simulink model "VCMGCM1962020b_v2"  (R2020b)
settings: Solver=FixedStepDiscrete  StartTime=0.0  StopTime=10.0  FixedStep=0.005  RelTol=1e-3  EnableMultiTasking=on
PreLoadFcn:
  | try, model_open; catch, disp('Error occurred while executing model pre-load callback: model_open.m'); disp('Please assure that the MATLAB working directory is set to the model directory before opening.'); end
InitFcn:
  | try, model_open; catch, end
undefined symbols (not defined in the file): Bridge, GCM, H, raptor_get_param_eval, raptor_get_safe_string, raptor_xcp_function
libraries: Blocks_lib x1165, Raptor_lib x665, simulink x62, VCM_lib x5
(part 18 of 23)

== system VCMGCM1962020b_v2/Fgnd/Sensors/CAN/Inverter/EM3_DCV/EM3PhCur ==
  DiagEnbl : Inport
  Enable : EnablePort
  CANRxFieldSingleFloat : Subsystem  AncestorBlock=Blocks_lib/CANRxField  mask(CANRxField){typ='double', custom=off, custom_nam='---', custom_units='---'}
      mask prompts: typ "Field Data Type"; custom "Use Custom Name and Units (instead of from .dbc file)"; custom_nam "Custom Name"; custom_units "Custom Units"
      mask help:
      | To be used with the raptor_can_rxmsg block.
      |
      | By default, the field name/units will be inherited from the .dbc file. For Custom Name or Units, check the checkbox. To use the inherited name/units in the custom name/units, use the string '---' to inhereit. For example, to simply add a prefix, the custom name would be something like 'prefix_---'.
      mask init: same as VCMGCM1962020b_v2/Fgnd/Sensors/CAN/Inverter/EM2_InvTemp/EM2InvTemp/CANRxFieldSingleFloat
      mask Callback custom:
      | raptor_set_param_enable(gcb, 'custom_nam', strcmp(get_param(gcb, 'custom'), 'on'));
      | raptor_set_param_enable(gcb, 'custom_units', strcmp(get_param(gcb, 'custom'), 'on'));
      mask Display:
      | disp(['CAN Rx: Field\n' nam '\n' units ', ' typ]);
      | 
      | port_label('input', 1, 'In');
  CANRxMsgStatus : Blocks_lib/CANRxMsgStatus  samptime=samptime  custom=on  custom_nam='EM_PhaseA'  msgnam=EM_PhaseA
  Header : Blocks_lib/Header  width=Landscape  addtext=''
  raptor_can_rxmsg1 : Raptor_lib/CAN/raptor_can_rxmsg  canDefinition=struct('dbcFile', '20220526e_emDrive_NodeID_0x01.dbc','message', 'EM3','comment', '40ms','signals', {{'EM3_InverterDcV','EM3_PhaseAmpsRms'}},'enabled', [ 0 1;],'scaled', [ 1 1;],'canBus', 'bus','messageID', [ 897;],'idMask', [ 536870911;],'payloadMask', [],'payloadValue', [],'period', [ 0;],'mailbox', '''''','queueSize', [ 1;],'label', [ 1;],'ver', [ 2;],'showID', [ 0;],'showRaw', [ 0;],'fill', [ 0;],'editID', [ 0;],'signalOrder', [ 1;],'signalAscDes', [ 1;])  canBus=bus  mailbox=''  payloadMask=[]  payloadValue=[]  idMask=hex2dec('1FFFFFFF')  queueSize=1  showID=0  label=1  fill=0  id=897  showRaw=0  showAge=1  signalOrder=1  signalInfo={{struct('Name', 'EM3_InverterDcV','Startbit', [ 0;],'SignalSize', [ 32;],'ByteOrder', 'LittleEndian','ValueType', 'FLOAT32','Class', 'single','Signed', [ 1;],'Factor', [ 1;],'Offset', [ 0;],'Min', [ 0;],'Max', [ 0;],'Units', 'V','Comment', 'HW_Monitor__UDC','StartBit', [ 0;]),struct('Name', 'EM3_PhaseAmpsRms','Startbit', [ 0;],'SignalSize', [ 32;],'ByteOrder', 'LittleEndian','ValueType', 'FLOAT32','Class', 'single','Signed', [ 1;],'Factor', [ 1;],'Offset', [ 0;],'Min', [ 0;],'Max', [ 0;],'Units', 'A','Comment', 'HW_Monitor__Phase_Current','StartBit', [ 32;])}}
      settings: SourceProductName=Raptor
  MsgVld : Outport
  Out2 : Outport  Port=2
  wires:
  raptor_can_rxmsg1/2 -> CANRxFieldSingleFloat/1(In)  "EM3_PhaseAmpsRms"
  raptor_can_rxmsg1/1 -> CANRxMsgStatus/2  "Age"
  DiagEnbl/1 -> CANRxMsgStatus/1
  CANRxFieldSingleFloat/1(Out) -> Out2/1
  CANRxMsgStatus/1 -> MsgVld/1

== system VCMGCM1962020b_v2/Fgnd/Sensors/CAN/Inverter/EM4_Spd/EM4Spd ==
  note: TBC: This logic is to get around an issue with a divide by a very small number, which is not recognized as zero
  DiagEnbl : Inport
  Enable : EnablePort
  Abs : Abs
  Bus Creator : BusCreator  Inputs=2
  Bus Selector : BusSelector  OutputSignals=EM4_SpdActVld [Bool],EM4_SpdAct [rpm]
  CANRxFieldSingleFloat : Subsystem  AncestorBlock=Blocks_lib/CANRxField  mask(CANRxField){typ='double', custom=off, custom_nam='---', custom_units='---'}
      mask prompts: typ "Field Data Type"; custom "Use Custom Name and Units (instead of from .dbc file)"; custom_nam "Custom Name"; custom_units "Custom Units"
      mask help:
      | To be used with the raptor_can_rxmsg block.
      |
      | By default, the field name/units will be inherited from the .dbc file. For Custom Name or Units, check the checkbox. To use the inherited name/units in the custom name/units, use the string '---' to inhereit. For example, to simply add a prefix, the custom name would be something like 'prefix_---'.
      mask init: same as VCMGCM1962020b_v2/Fgnd/Sensors/CAN/Inverter/EM2_InvTemp/EM2InvTemp/CANRxFieldSingleFloat
      mask Callback custom:
      | raptor_set_param_enable(gcb, 'custom_nam', strcmp(get_param(gcb, 'custom'), 'on'));
      | raptor_set_param_enable(gcb, 'custom_units', strcmp(get_param(gcb, 'custom'), 'on'));
      mask Display:
      | disp(['CAN Rx: Field\n' nam '\n' units ', ' typ]);
      | 
      | port_label('input', 1, 'In');
  CANRxMsgStatus : Blocks_lib/CANRxMsgStatus  samptime=samptime  custom=on  custom_nam='EM4_Spd'  msgnam=EM4_Spd
  Compare To Constant : simulink/Logic and Bit Operations/Compare To Constant  relop=>  const=1  OutDataTypeStr=boolean
  Constant : Constant  Value=0
  Header : Blocks_lib/Header  width=Landscape  addtext=''
  Switch : Switch  Criteria=u2 > Threshold
  raptor_can_rxmsg1 : Raptor_lib/CAN/raptor_can_rxmsg  canDefinition=struct('dbcFile', '20220526e_emDrive_NodeID_0x01.dbc','message', 'EM4','comment', '20ms','signals', {{'EM4_SpdAct','EM4_TorqAct'}},'enabled', [ 1 0;],'scaled', [ 1 1;],'canBus', 'bus','messageID', [ 641;],'idMask', [ 536870911;],'payloadMask', [],'payloadValue', [],'period', [ 0;],'mailbox', '''''','queueSize', [ 1;],'label', [ 1;],'ver', [ 2;],'showID', [ 0;],'showRaw', [ 0;],'fill', [ 0;],'editID', [ 0;],'signalOrder', [ 1;],'signalAscDes', [ 1;])  canBus=bus  mailbox=''  payloadMask=[]  payloadValue=[]  idMask=hex2dec('1FFFFFFF')  queueSize=1  showID=0  label=1  fill=0  id=641  showRaw=0  showAge=1  signalOrder=1  signalInfo={{struct('Name', 'EM4_TorqAct','Startbit', [ 0;],'SignalSize', [ 32;],'ByteOrder', 'LittleEndian','ValueType', 'FLOAT32','Class', 'single','Signed', [ 1;],'Factor', [ 1;],'Offset', [ 0;],'Min', [ 0;],'Max', [ 0;],'Units', 'Nm','Comment', 'Ctrl_Gen_Stat__Tact','StartBit', [ 0;]),struct('Name', 'EM4_SpdAct','Startbit', [ 0;],'SignalSize', [ 32;],'ByteOrder', 'LittleEndian','ValueType', 'FLOAT32','Class', 'single','Signed', [ 1;],'Factor', [ 1;],'Offset', [ 0;],'Min', [ 0;],'Max', [ 0;],'Units', 'rpm','Comment', 'Ctrl_Gen_Stat__RPMact','StartBit', [ 32;])}}
      settings: SourceProductName=Raptor
  MsgVld : Outport
  Out2 : Outport  Port=2
  wires:
  raptor_can_rxmsg1/2 -> CANRxFieldSingleFloat/1(In)  "EM4_SpdAct"
  raptor_can_rxmsg1/1 -> CANRxMsgStatus/2  "Age"
  DiagEnbl/1 -> CANRxMsgStatus/1
  CANRxMsgStatus/1 -> MsgVld/1
  Constant/1 -> Switch/3
  Abs/1 -> Compare To Constant/1
  Compare To Constant/1 -> Switch/2
  CANRxFieldSingleFloat/1(Out) -> Bus Selector/1
  Bus Selector/2 -> Switch/1, Abs/1  "<EM4_SpdAct [rpm]>"
  Bus Creator/1 -> Out2/1  "EM4_SpdAct"
  Bus Selector/1 -> Bus Creator/1  "<EM4_SpdActVld [Bool]>"
  Switch/1 -> Bus Creator/2  "EM4_SpdAct [rpm]"

== system VCMGCM1962020b_v2/Fgnd/Sensors/CAN/Inverter/EM4_Spd/EM4Torq ==
  DiagEnbl : Inport
  Enable : EnablePort
  CANRxFieldSingleFloat : Subsystem  AncestorBlock=Blocks_lib/CANRxField  mask(CANRxField){typ='double', custom=off, custom_nam='---', custom_units='---'}
      mask prompts: typ "Field Data Type"; custom "Use Custom Name and Units (instead of from .dbc file)"; custom_nam "Custom Name"; custom_units "Custom Units"
      mask help:
      | To be used with the raptor_can_rxmsg block.
      |
      | By default, the field name/units will be inherited from the .dbc file. For Custom Name or Units, check the checkbox. To use the inherited name/units in the custom name/units, use the string '---' to inhereit. For example, to simply add a prefix, the custom name would be something like 'prefix_---'.
      mask init: same as VCMGCM1962020b_v2/Fgnd/Sensors/CAN/Inverter/EM2_InvTemp/EM2InvTemp/CANRxFieldSingleFloat
      mask Callback custom:
      | raptor_set_param_enable(gcb, 'custom_nam', strcmp(get_param(gcb, 'custom'), 'on'));
      | raptor_set_param_enable(gcb, 'custom_units', strcmp(get_param(gcb, 'custom'), 'on'));
      mask Display:
      | disp(['CAN Rx: Field\n' nam '\n' units ', ' typ]);
      | 
      | port_label('input', 1, 'In');
  CANRxMsgStatus : Blocks_lib/CANRxMsgStatus  samptime=samptime  custom=on  custom_nam='EM4_Trq'  msgnam=EM4_Trq
  Header : Blocks_lib/Header  width=Landscape  addtext=''
  raptor_can_rxmsg1 : Raptor_lib/CAN/raptor_can_rxmsg  canDefinition=struct('dbcFile', '20220526e_emDrive_NodeID_0x01.dbc','message', 'EM4','comment', '20ms','signals', {{'EM4_SpdAct','EM4_TorqAct'}},'enabled', [ 0 1;],'scaled', [ 1 1;],'canBus', 'bus','messageID', [ 641;],'idMask', [ 536870911;],'payloadMask', [],'payloadValue', [],'period', [ 0;],'mailbox', '''''','queueSize', [ 1;],'label', [ 1;],'ver', [ 2;],'showID', [ 0;],'showRaw', [ 0;],'fill', [ 0;],'editID', [ 0;],'signalOrder', [ 1;],'signalAscDes', [ 1;])  canBus=bus  mailbox=''  payloadMask=[]  payloadValue=[]  idMask=hex2dec('1FFFFFFF')  queueSize=1  showID=0  label=1  fill=0  id=641  showRaw=0  showAge=1  signalOrder=1  signalInfo={{struct('Name', 'EM4_TorqAct','Startbit', [ 0;],'SignalSize', [ 32;],'ByteOrder', 'LittleEndian','ValueType', 'FLOAT32','Class', 'single','Signed', [ 1;],'Factor', [ 1;],'Offset', [ 0;],'Min', [ 0;],'Max', [ 0;],'Units', 'Nm','Comment', 'Ctrl_Gen_Stat__Tact','StartBit', [ 0;]),struct('Name', 'EM4_SpdAct','Startbit', [ 0;],'SignalSize', [ 32;],'ByteOrder', 'LittleEndian','ValueType', 'FLOAT32','Class', 'single','Signed', [ 1;],'Factor', [ 1;],'Offset', [ 0;],'Min', [ 0;],'Max', [ 0;],'Units', 'rpm','Comment', 'Ctrl_Gen_Stat__RPMact','StartBit', [ 32;])}}
      settings: SourceProductName=Raptor
  MsgVld : Outport
  Out2 : Outport  Port=2
  wires:
  raptor_can_rxmsg1/2 -> CANRxFieldSingleFloat/1(In)  "EM4_TorqAct"
  raptor_can_rxmsg1/1 -> CANRxMsgStatus/2  "Age"
  DiagEnbl/1 -> CANRxMsgStatus/1
  CANRxFieldSingleFloat/1(Out) -> Out2/1
  CANRxMsgStatus/1 -> MsgVld/1

== system VCMGCM1962020b_v2/Fgnd/Sensors/CAN/Other/A//C Compressor/ACCSTATUS2 ==
  DiagEnbl : Inport
  Bus Creator : BusCreator  Inputs=7
  CANRxField : Blocks_lib/CANRxField  typ='boolean'  custom=on  custom_nam=[nam '---']  custom_units='---'
  CANRxField1 : Blocks_lib/CANRxField  typ='boolean'  custom=on  custom_nam=[nam '---']  custom_units='---'
  CANRxField2 : Blocks_lib/CANRxField  typ='boolean'  custom=on  custom_nam=[nam '---']  custom_units='---'
  CANRxField3 : Blocks_lib/CANRxField  typ='double'  custom=on  custom_nam=[nam '---']  custom_units='---'
  CANRxField4 : Blocks_lib/CANRxField  typ='double'  custom=on  custom_nam=[nam '---']  custom_units='---'
  CANRxField5 : Blocks_lib/CANRxField  typ='double'  custom=on  custom_nam=[nam '---']  custom_units='---'
  CANRxMsgStatus : Blocks_lib/CANRxMsgStatus  samptime=samptime  custom=on  custom_nam=[nam '---']  msgnam=ACCSTATUS2
  Header : Blocks_lib/Header  width=Landscape  addtext=''
  raptor_can_rxmsg : Raptor_lib/CAN/raptor_can_rxmsg  canDefinition=struct('dbcFile', 'ACCompressor_MitsubishiEV36BNx.dbc','message', 'STATUS2','comment', '','signals', {{'IGBTTempV','HVInputV','BoardTempV','BoardTemp','HVInput','IGBTTemp'}},'enabled', [ 1 1 1 1 1 1;],'scaled', [ 1 1 1 1 1 1;],'canBus', 'bus','messageID', [ 141598791;],'idMask', [ 536870911;],'payloadMask', [],'payloadValue', [],'period', [ 0;],'mailbox', '''''','queueSize', [ 1;],'label', [ 1;],'ver', [ 2;],'showID', [ 0;],'showRaw', [ 0;],'fill', [ 0;],'editID', [ 0;],'signalOrder', [ 3;],'signalAscDes', [ 1;])  canBus=bus  mailbox=''  payloadMask=[]  payloadValue=[]  idMask=hex2dec('1FFFFFFF')  queueSize=1  showID=0  label=1  fill=0  id=141598791  showRaw=0  showAge=1  signalOrder=3  signalInfo={{struct('Name', 'IGBTTempV','Startbit', [ 0;],'SignalSize', [ 1;],'ByteOrder', 'LittleEndian','ValueType', 'UNSIGNED','Class', 'uint8','Signed', [ 0;],'Factor', [ 1;],'Offset', [ 0;],'Min', [ 0;],'Max', [ 1;],'Units', '','Comment', '','StartBit', [ 2;]),struct('Name', 'HVInputV','Startbit', [ 0;],'SignalSize', [ 1;],'ByteOrder', 'LittleEndian','ValueType', 'UNSIGNED','Class', 'uint8','Signed', [ 0;],'Factor', [ 1;],'Offset', [ 0;],'Min', [ 0;],'Max', [ 1;],'Units', '','Comment', '','StartBit', [ 1;]),struct('Name', 'BoardTempV','Startbit', [ 0;],'SignalSize', [ 1;],'ByteOrder', 'LittleEndian','ValueType', 'UNSIGNED','Class', 'uint8','Signed', [ 0;],'Factor', [ 1;],'Offset', [ 0;],'Min', [ 0;],'Max', [ 1;],'Units', '','Comment', '','StartBit', [ 0;]),struct('Name', 'BoardTemp','Startbit', [ 0;],'SignalSize', [ 8;],'ByteOrder', 'LittleEndian','ValueType', 'UNSIGNED','Class', 'uint8','Signed', [ 0;],'Factor', [ 1;],'Offset', [ -40;],'Min', [ -40;],'Max', [ 215;],'Units', 'degC','Comment', '','StartBit', [ 8;]),struct('Name', 'HVInput','Startbit', [ 0;],'SignalSize', [ 8;],'ByteOrder', 'LittleEndian','ValueType', 'UNSIGNED','Class', 'uint8','Signed', [ 0;],'Factor', [ 4;],'Offset', [ 0;],'Min', [ 0;],'Max', [ 1020;],'Units', 'Volts','Comment', '','StartBit', [ 16;]),struct('Name', 'IGBTTemp','Startbit', [ 0;],'SignalSize', [ 8;],'ByteOrder', 'LittleEndian','ValueType', 'UNSIGNED','Class', 'uint8','Signed', [ 0;],'Factor', [ 1;],'Offset', [ -40;],'Min', [ -40;],'Max', [ 215;],'Units', 'degC','Comment', '','StartBit', [ 24;])}}
      settings: SourceProductName=Raptor
  Data : Outport  VectorParamsAs1DForOutWhenUnconnected=off
  wires:
  raptor_can_rxmsg/1 -> CANRxMsgStatus/2  "Age"
  DiagEnbl/1 -> CANRxMsgStatus/1
  CANRxMsgStatus/1 -> Bus Creator/1
  CANRxField/1 -> Bus Creator/2
  raptor_can_rxmsg/3 -> CANRxField1/1  "HVInputV"
  raptor_can_rxmsg/2 -> CANRxField/1  "IGBTTempV"
  Bus Creator/1 -> Data/1  "MsgName"
  raptor_can_rxmsg/4 -> CANRxField2/1  "BoardTempV"
  raptor_can_rxmsg/5 -> CANRxField3/1  "BoardTemp"
  raptor_can_rxmsg/6 -> CANRxField4/1  "HVInput"
  raptor_can_rxmsg/7 -> CANRxField5/1  "IGBTTemp"
  CANRxField1/1 -> Bus Creator/3
  CANRxField2/1 -> Bus Creator/4
  CANRxField3/1 -> Bus Creator/5
  CANRxField4/1 -> Bus Creator/6
  CANRxField5/1 -> Bus Creator/7

== system VCMGCM1962020b_v2/Fgnd/Sensors/CAN/Other/A//C Compressor/MsgName ==
  DiagEnbl : Inport
  Bus Creator : BusCreator  Inputs=10
  CANRxField{,2..4} (4 alike) : Blocks_lib/CANRxField  typ='boolean'  custom=on  custom_nam=[nam '---']  custom_units='---'
  CANRxField1 : Blocks_lib/CANRxField  typ='uint8'  custom=on  custom_nam=[nam '---']  custom_units='---'
  CANRxField5 : Blocks_lib/CANRxField  typ='double'  custom=on  custom_nam=[nam '---']  custom_units='---'
  CANRxField6 : Blocks_lib/CANRxField  typ='double'  custom=on  custom_nam=[nam '---']  custom_units='---'
  CANRxField7 : Blocks_lib/CANRxField  typ='double'  custom=on  custom_nam=[nam '---']  custom_units='---'
  CANRxField8 : Blocks_lib/CANRxField  typ='uint8'  custom=on  custom_nam=[nam '---']  custom_units='---'
  CANRxMsgStatus : Blocks_lib/CANRxMsgStatus  samptime=samptime  custom=on  custom_nam=[nam '---']  msgnam=ACCSTATUS1
  Header : Blocks_lib/Header  width=Landscape  addtext=''
  raptor_can_rxmsg : Raptor_lib/CAN/raptor_can_rxmsg  canDefinition=struct('dbcFile', 'ACCompressor_MitsubishiEV36BNx.dbc','message', 'STATUS1','comment', '','signals', {{'ElecCurrV','Stat','ElecPwrV','SpdIncrReq','SpdV','ElecPwr','Spd','ElecCurr','FltStat'}},'enabled', [ 1 1 1 1 1 1 1 1 1;],'scaled', [ 1 1 1 1 1 1 1 1 1;],'canBus', 'bus','messageID', [ 141074503;],'idMask', [ 536870911;],'payloadMask', [],'payloadValue', [],'period', [ 0;],'mailbox', '''''','queueSize', [ 1;],'label', [ 1;],'ver', [ 2;],'showID', [ 0;],'showRaw', [ 0;],'fill', [ 0;],'editID', [ 0;],'signalOrder', [ 3;],'signalAscDes', [ 1;])  canBus=bus  mailbox=''  payloadMask=[]  payloadValue=[]  idMask=hex2dec('1FFFFFFF')  queueSize=1  showID=0  label=1  fill=0  id=141074503  showRaw=0  showAge=1  signalOrder=3  signalInfo={{struct('Name', 'ElecCurrV','Startbit', [ 0;],'SignalSize', [ 1;],'ByteOrder', 'LittleEndian','ValueType', 'UNSIGNED','Class', 'uint8','Signed', [ 0;],'Factor', [ 1;],'Offset', [ 0;],'Min', [ 0;],'Max', [ 1;],'Units', '','Comment', '','StartBit', [ 7;]),struct('Name', 'Stat','Startbit', [ 0;],'SignalSize', [ 4;],'ByteOrder', 'LittleEndian','ValueType', 'UNSIGNED','Class', 'uint8','Signed', [ 0;],'Factor', [ 1;],'Offset', [ 0;],'Min', [ 0;],'Max', [ 2;],'Units', '','Comment', '','StartBit', [ 3;]),struct('Name', 'ElecPwrV','Startbit', [ 0;],'SignalSize', [ 1;],'ByteOrder', 'LittleEndian','ValueType', 'UNSIGNED','Class', 'uint8','Signed', [ 0;],'Factor', [ 1;],'Offset', [ 0;],'Min', [ 0;],'Max', [ 0;],'Units', '','Comment', '','StartBit', [ 2;]),struct('Name', 'SpdIncrReq','Startbit', [ 0;],'SignalSize', [ 1;],'ByteOrder', 'LittleEndian','ValueType', 'UNSIGNED','Class', 'uint8','Signed', [ 0;],'Factor', [ 1;],'Offset', [ 0;],'Min', [ 0;],'Max', [ 1;],'Units', '','Comment', '','StartBit', [ 1;]),struct('Name', 'SpdV','Startbit', [ 0;],'SignalSize', [ 1;],'ByteOrder', 'LittleEndian','ValueType', 'UNSIGNED','Class', 'uint8','Signed', [ 0;],'Factor', [ 1;],'Offset', [ 0;],'Min', [ 0;],'Max', [ 1;],'Units', '','Comment', '','StartBit', [ 0;]),struct('Name', 'ElecPwr','Startbit', [ 0;],'SignalSize', [ 8;],'ByteOrder', 'LittleEndian','ValueType', 'UNSIGNED','Class', 'uint8','Signed', [ 0;],'Factor', [ 40;],'Offset', [ 0;],'Min', [ 0;],'Max', [ 10200;],'Units', 'Watts','Comment', '','StartBit', [ 8;]),struct('Name', 'Spd','Startbit', [ 0;],'SignalSize', [ 14;],'ByteOrder', 'BigEndian','ValueType', 'UNSIGNED','Class', 'uint16','Signed', [ 0;],'Factor', [ 1;],'Offset', [ 0;],'Min', [ 0;],'Max', [ 16383;],'Units', 'RPM','Comment', '','StartBit', [ 24;]),struct('Name', 'ElecCurr','Startbit', [ 0;],'SignalSize', [ 8;],'ByteOrder', 'LittleEndian','ValueType', 'UNSIGNED','Class', 'uint8','Signed', [ 0;],'Factor', [ 0.2;],'Offset', [ 0;],'Min', [ 0;],'Max', [ 51;],'Units', 'Amps','Comment', '','StartBit', [ 32;]),struct('Name', 'FltStat','Startbit', [ 0;],'SignalSize', [ 4;],'ByteOrder', 'LittleEndian','ValueType', 'UNSIGNED','Class', 'uint8','Signed', [ 0;],'Factor', [ 1;],'Offset', [ 0;],'Min', [ 0;],'Max', [ 6;],'Units', '','Comment', '','StartBit', [ 40;])}}
      settings: SourceProductName=Raptor
  Data : Outport  VectorParamsAs1DForOutWhenUnconnected=off
  wires:
  raptor_can_rxmsg/1 -> CANRxMsgStatus/2  "Age"
  DiagEnbl/1 -> CANRxMsgStatus/1
  CANRxMsgStatus/1 -> Bus Creator/1
  CANRxField/1 -> Bus Creator/2
  raptor_can_rxmsg/3 -> CANRxField1/1  "Stat"
  raptor_can_rxmsg/2 -> CANRxField/1  "ElecCurrV"
  Bus Creator/1 -> Data/1  "MsgName"
  raptor_can_rxmsg/4 -> CANRxField2/1  "ElecPwrV"
  raptor_can_rxmsg/5 -> CANRxField3/1  "SpdIncrReq"
  raptor_can_rxmsg/6 -> CANRxField4/1  "SpdV"
  raptor_can_rxmsg/7 -> CANRxField5/1  "ElecPwr"
  raptor_can_rxmsg/8 -> CANRxField6/1  "Spd"
  raptor_can_rxmsg/9 -> CANRxField7/1  "ElecCurr"
  raptor_can_rxmsg/10 -> CANRxField8/1  "FltStat"
  CANRxField1/1 -> Bus Creator/3
  CANRxField2/1 -> Bus Creator/4
  CANRxField3/1 -> Bus Creator/5
  CANRxField4/1 -> Bus Creator/6
  CANRxField5/1 -> Bus Creator/7
  CANRxField6/1 -> Bus Creator/8
  CANRxField7/1 -> Bus Creator/9
  CANRxField8/1 -> Bus Creator/10

== system VCMGCM1962020b_v2/Fgnd/Sensors/CAN/Other/BCM/BCMAMB ==
  DiagEnbl : Inport
  Bus Creator : BusCreator  Inputs=3
  CANRxField : Blocks_lib/CANRxField  typ='double'  custom=off  custom_nam=[nam '---']  custom_units='---'
  CANRxField1 : Blocks_lib/CANRxField  typ='double'  custom=off  custom_nam=[nam '---']  custom_units='---'
  CANRxMsgStatus : Blocks_lib/CANRxMsgStatus  samptime=samptime  custom=on  custom_nam=[nam '---']  msgnam=BCMAMB
  Header : Blocks_lib/Header  width=Landscape  addtext=''
  raptor_can_rxmsg : Raptor_lib/CAN/raptor_can_rxmsg  canDefinition=struct('dbcFile', 'BCM_dbc_file_rev_9.1.dbc','message', 'AMB','comment', '','signals', {{'Amb_Air_Temp','Cab_Temp'}},'enabled', [ 1 1;],'scaled', [ 1 1;],'canBus', 'bus','messageID', [ 419362081;],'idMask', [ 536870911;],'payloadMask', [],'payloadValue', [],'period', [ 0;],'mailbox', '[]','queueSize', [ 1;],'label', [ 1;],'ver', [ 2;],'showID', [ 0;],'showRaw', [ 0;],'fill', [ 0;],'editID', [ 0;],'signalOrder', [ 3;],'signalAscDes', [ 1;])  canBus=bus  mailbox=[]  payloadMask=[]  payloadValue=[]  idMask=hex2dec('1FFFFFFF')  queueSize=1  showID=0  label=1  fill=0  id=419362081  showRaw=0  showAge=1  signalOrder=3  signalInfo={{struct('Name', 'Amb_Air_Temp','Startbit', [ 0;],'SignalSize', [ 16;],'ByteOrder', 'LittleEndian','ValueType', 'UNSIGNED','Class', 'uint16','Signed', [ 0;],'Factor', [ 0.03125;],'Offset', [ -273;],'Min', [ -273;],'Max', [ 1734.97;],'Units', 'C','Comment', '','StartBit', [ 24;]),struct('Name', 'Cab_Temp','Startbit', [ 0;],'SignalSize', [ 16;],'ByteOrder', 'LittleEndian','ValueType', 'UNSIGNED','Class', 'uint16','Signed', [ 0;],'Factor', [ 0.03125;],'Offset', [ -273;],'Min', [ -273;],'Max', [ 1734.97;],'Units', 'C','Comment', '','StartBit', [ 8;])}}
      settings: SourceProductName=Raptor
  Data : Outport  VectorParamsAs1DForOutWhenUnconnected=off
  wires:
  raptor_can_rxmsg/3 -> CANRxField1/1  "Cab_Temp"
  Bus Creator/1 -> Data/1  "BCMAMB"
  raptor_can_rxmsg/2 -> CANRxField/1  "Amb_Air_Temp"
  CANRxMsgStatus/1 -> Bus Creator/1
  CANRxField/1 -> Bus Creator/2
  CANRxField1/1 -> Bus Creator/3
  DiagEnbl/1 -> CANRxMsgStatus/1
  raptor_can_rxmsg/1 -> CANRxMsgStatus/2  "Age"

== system VCMGCM1962020b_v2/Fgnd/Sensors/CAN/Other/BCM/BCMCab_Mssg1 ==
  DiagEnbl : Inport
  Bus Creator : BusCreator  Inputs=2
  CANRxField : Blocks_lib/CANRxField  typ='uint8'  custom=off  custom_nam=[nam '---']  custom_units='---'
  CANRxMsgStatus : Blocks_lib/CANRxMsgStatus  samptime=samptime  custom=on  custom_nam=[nam '---']  msgnam=BCMCab_Mssg1
  Header : Blocks_lib/Header  width=Landscape  addtext=''
  raptor_can_rxmsg : Raptor_lib/CAN/raptor_can_rxmsg  canDefinition=struct('dbcFile', 'BCM_dbc_file_rev_9.1.dbc','message', 'Cab_Mssg1','comment', '','signals', {{'Seatbelt_Switch'}},'enabled', [ 1;],'scaled', [ 1;],'canBus', 'bus','messageID', [ 417333281;],'idMask', [ 536870911;],'payloadMask', [],'payloadValue', [],'period', [ 0;],'mailbox', '[]','queueSize', [ 1;],'label', [ 1;],'ver', [ 2;],'showID', [ 0;],'showRaw', [ 0;],'fill', [ 0;],'editID', [ 0;],'signalOrder', [ 3;],'signalAscDes', [ 1;])  canBus=bus  mailbox=[]  payloadMask=[]  payloadValue=[]  idMask=hex2dec('1FFFFFFF')  queueSize=1  showID=0  label=1  fill=0  id=417333281  showRaw=0  showAge=1  signalOrder=3  signalInfo={{struct('Name', 'Seatbelt_Switch','Startbit', [ 0;],'SignalSize', [ 2;],'ByteOrder', 'LittleEndian','ValueType', 'UNSIGNED','Class', 'uint8','Signed', [ 0;],'Factor', [ 1;],'Offset', [ 0;],'Min', [ 0;],'Max', [ 3;],'Units', 'enum','Comment', '','StartBit', [ 30;])}}
      settings: SourceProductName=Raptor
  Data : Outport  VectorParamsAs1DForOutWhenUnconnected=off
  wires:
  Bus Creator/1 -> Data/1  "BCMCab_Mssg1"
  raptor_can_rxmsg/2 -> CANRxField/1  "Seatbelt_Switch"
  CANRxMsgStatus/1 -> Bus Creator/1
  CANRxField/1 -> Bus Creator/2
  DiagEnbl/1 -> CANRxMsgStatus/1
  raptor_can_rxmsg/1 -> CANRxMsgStatus/2  "Age"

== system VCMGCM1962020b_v2/Fgnd/Sensors/CAN/Other/BCM/CCVS1_BCM ==
  DiagEnbl : Inport
  Bus Creator : BusCreator  Inputs=2
  CANRxField : Blocks_lib/CANRxField  typ='uint8'  custom=off  custom_nam=[nam '---']  custom_units='---'
  CANRxMsgStatus : Blocks_lib/CANRxMsgStatus  samptime=samptime  custom=off  custom_nam=[nam '---']  msgnam=CCVS1_BCM
  Header : Blocks_lib/Header  width=Landscape  addtext=''
  raptor_can_rxmsg : Raptor_lib/CAN/raptor_can_rxmsg  canDefinition=struct('dbcFile', 'BCM_dbc_file_rev_9.1.dbc','message', 'CCVS1_BCM','comment', '','signals', {{'Parking_Brak_Switch'}},'enabled', [ 1;],'scaled', [ 1;],'canBus', 'bus','messageID', [ 419361057;],'idMask', [ 536870911;],'payloadMask', [],'payloadValue', [],'period', [ 0;],'mailbox', '[]','queueSize', [ 1;],'label', [ 1;],'ver', [ 2;],'showID', [ 0;],'showRaw', [ 0;],'fill', [ 0;],'editID', [ 0;],'signalOrder', [ 3;],'signalAscDes', [ 1;])  canBus=bus  mailbox=[]  payloadMask=[]  payloadValue=[]  idMask=hex2dec('1FFFFFFF')  queueSize=1  showID=0  label=1  fill=0  id=419361057  showRaw=0  showAge=1  signalOrder=3  signalInfo={{struct('Name', 'Parking_Brak_Switch','Startbit', [ 0;],'SignalSize', [ 2;],'ByteOrder', 'LittleEndian','ValueType', 'UNSIGNED','Class', 'uint8','Signed', [ 0;],'Factor', [ 1;],'Offset', [ 0;],'Min', [ 0;],'Max', [ 3;],'Units', 'enum','Comment', '','StartBit', [ 0;])}}
      settings: SourceProductName=Raptor
  Data : Outport  VectorParamsAs1DForOutWhenUnconnected=off
  wires:
  Bus Creator/1 -> Data/1  "CCVS1_BCM"
  raptor_can_rxmsg/2 -> CANRxField/1  "Parking_Brak_Switch"
  CANRxMsgStatus/1 -> Bus Creator/1
  CANRxField/1 -> Bus Creator/2
  DiagEnbl/1 -> CANRxMsgStatus/1
  raptor_can_rxmsg/1 -> CANRxMsgStatus/2  "Age"

== system VCMGCM1962020b_v2/Fgnd/Sensors/CAN/Other/BCM1/DisplayTG1 ==
  DiagEnbl : Inport
  Bus Creator : BusCreator  Inputs=2
  CANRxField : Blocks_lib/CANRxField  typ='double'  custom=off  custom_nam=[nam '---']  custom_units='---'
  CANRxMsgStatus : Blocks_lib/CANRxMsgStatus  samptime=samptime  custom=on  custom_nam=[nam '---']  msgnam=DisplayTG1
  Header : Blocks_lib/Header  width=Landscape  addtext=''
  raptor_can_rxmsg : Raptor_lib/CAN/raptor_can_rxmsg  canDefinition=struct('dbcFile', 'Drivers_Disp_dbc_file_v5.0.dbc','message', 'TG1','comment', '','signals', {{'Trip_Reset'}},'enabled', [ 1;],'scaled', [ 1;],'canBus', 'bus','messageID', [ 417202430;],'idMask', [ 536870911;],'payloadMask', [],'payloadValue', [],'period', [ 0;],'mailbox', '[]','queueSize', [ 1;],'label', [ 1;],'ver', [ 2;],'showID', [ 0;],'showRaw', [ 0;],'fill', [ 0;],'editID', [ 0;],'signalOrder', [ 3;],'signalAscDes', [ 1;])  canBus=bus  mailbox=[]  payloadMask=[]  payloadValue=[]  idMask=hex2dec('1FFFFFFF')  queueSize=1  showID=0  label=1  fill=0  id=417202430  showRaw=0  showAge=1  signalOrder=3  signalInfo={{struct('Name', 'Trip_Reset','Startbit', [ 0;],'SignalSize', [ 2;],'ByteOrder', 'LittleEndian','ValueType', 'UNSIGNED','Class', 'uint8','Signed', [ 0;],'Factor', [ 1;],'Offset', [ 0;],'Min', [ 0;],'Max', [ 3;],'Units', 'enum','Comment', '','StartBit', [ 0;])}}
      settings: SourceProductName=Raptor
  Data : Outport  VectorParamsAs1DForOutWhenUnconnected=off
  wires:
  Bus Creator/1 -> Data/1  "DisplayTG1"
  raptor_can_rxmsg/2 -> CANRxField/1  "Trip_Reset"
  CANRxMsgStatus/1 -> Bus Creator/1
  CANRxField/1 -> Bus Creator/2
  DiagEnbl/1 -> CANRxMsgStatus/1
  raptor_can_rxmsg/1 -> CANRxMsgStatus/2  "Age"

== system VCMGCM1962020b_v2/Fgnd/Sensors/CAN/Other/Charge Port DC Voltage Sensor/cs_ivt_msg_result_voltage_ch1 ==
  DiagEnbl : Inport
  Bus Creator : BusCreator  Inputs=8
  CANRxField{,1,5..6} (4 alike) : Blocks_lib/CANRxField  typ='boolean'  custom=off  custom_nam='---'  custom_units='---'
  CANRxField2 : Blocks_lib/CANRxField  typ='double'  custom=off  custom_nam='---'  custom_units='---'
  CANRxField3 : Blocks_lib/CANRxField  typ='uint8'  custom=off  custom_nam='---'  custom_units='---'
  CANRxField4 : Blocks_lib/CANRxField  typ='uint8'  custom=off  custom_nam='---'  custom_units='---'
  CANRxMsgStatus : Blocks_lib/CANRxMsgStatus  samptime=samptime  custom=off  custom_nam='Name'  msgnam=cs_ivt_msg_result_voltage_ch1
  Header : Blocks_lib/Header  width=Landscape  addtext=''
  raptor_can_rxmsg : Raptor_lib/CAN/raptor_can_rxmsg  canDefinition=struct('dbcFile', 'ivt_current_sensor.dbc','message', 'cs_ivt_msg_result_voltage_ch1','comment', '','signals', {{'result_volt_ch1_channel_error','result_volt_ch1_meas_error','result_volt_ch1_meas_value','result_volt_ch1_msg_count','result_volt_ch1_mux_id','result_volt_ch1_system_error','result_volt_ch1_ocs'}},'enabled', [ 1 1 1 1 1 1 1;],'scaled', [ 1 1 1 1 1 1 1;],'canBus', 'bus','messageID', [ 1314;],'idMask', [ 536870911;],'payloadMask', [],'payloadValue', [],'period', [ 0;],'mailbox', '''''','queueSize', [ 1;],'label', [ 1;],'ver', [ 2;],'showID', [ 0;],'showRaw', [ 0;],'fill', [ 0;],'editID', [ 0;],'signalOrder', [ 3;],'signalAscDes', [ 1;])  canBus=bus  mailbox=''  payloadMask=[]  payloadValue=[]  idMask=hex2dec('1FFFFFFF')  queueSize=1  showID=0  label=1  fill=0  id=1314  showRaw=0  showAge=1  signalOrder=3  signalInfo={{struct('Name', 'result_volt_ch1_channel_error','Startbit', [ 0;],'SignalSize', [ 1;],'ByteOrder', 'BigEndian','ValueType', 'UNSIGNED','Class', 'uint8','Signed', [ 0;],'Factor', [ 1;],'Offset', [ 0;],'Min', [ 0;],'Max', [ 1;],'Units', '','Comment', '','StartBit', [ 13;]),struct('Name', 'result_volt_ch1_meas_error','Startbit', [ 0;],'SignalSize', [ 1;],'ByteOrder', 'BigEndian','ValueType', 'UNSIGNED','Class', 'uint8','Signed', [ 0;],'Factor', [ 1;],'Offset', [ 0;],'Min', [ 0;],'Max', [ 1;],'Units', '','Comment', '','StartBit', [ 14;]),struct('Name', 'result_volt_ch1_meas_value','Startbit', [ 0;],'SignalSize', [ 32;],'ByteOrder', 'BigEndian','ValueType', 'SIGNED','Class', 'int32','Signed', [ 1;],'Factor', [ 1;],'Offset', [ 0;],'Min', [ -2147483648;],'Max', [ 2147483647;],'Units', '','Comment', '','StartBit', [ 40;]),struct('Name', 'result_volt_ch1_msg_count','Startbit', [ 0;],'SignalSize', [ 4;],'ByteOrder', 'BigEndian','ValueType', 'UNSIGNED','Class', 'uint8','Signed', [ 0;],'Factor', [ 1;],'Offset', [ 0;],'Min', [ 0;],'Max', [ 15;],'Units', '','Comment', '','StartBit', [ 8;]),struct('Name', 'result_volt_ch1_mux_id','Startbit', [ 0;],'SignalSize', [ 8;],'ByteOrder', 'BigEndian','ValueType', 'UNSIGNED','Class', 'uint8','Signed', [ 0;],'Factor', [ 1;],'Offset', [ 0;],'Min', [ 0;],'Max', [ 255;],'Units', '','Comment', '','StartBit', [ 0;]),struct('Name', 'result_volt_ch1_system_error','Startbit', [ 0;],'SignalSize', [ 1;],'ByteOrder', 'BigEndian','ValueType', 'UNSIGNED','Class', 'uint8','Signed', [ 0;],'Factor', [ 1;],'Offset', [ 0;],'Min', [ 0;],'Max', [ 1;],'Units', '','Comment', '','StartBit', [ 15;]),struct('Name', 'result_volt_ch1_ocs','Startbit', [ 0;],'SignalSize', [ 1;],'ByteOrder', 'BigEndian','ValueType', 'UNSIGNED','Class', 'uint8','Signed', [ 0;],'Factor', [ 1;],'Offset', [ 0;],'Min', [ 0;],'Max', [ 1;],'Units', '','Comment', '','StartBit', [ 12;])}}
      settings: SourceProductName=Raptor
  Data : Outport  VectorParamsAs1DForOutWhenUnconnected=off
  wires:
  raptor_can_rxmsg/1 -> CANRxMsgStatus/2  "Age"
  DiagEnbl/1 -> CANRxMsgStatus/1
  CANRxMsgStatus/1 -> Bus Creator/1
  Bus Creator/1 -> Data/1  "cs_ivt_msg_result_voltage_ch1"
  raptor_can_rxmsg/2 -> CANRxField/1  "result_volt_ch1_channel_error"
  raptor_can_rxmsg/3 -> CANRxField1/1  "result_volt_ch1_meas_error"
  raptor_can_rxmsg/4 -> CANRxField2/1  "result_volt_ch1_meas_value"
  raptor_can_rxmsg/5 -> CANRxField3/1  "result_volt_ch1_msg_count"
  raptor_can_rxmsg/8 -> CANRxField6/1  "result_volt_ch1_ocs"
  raptor_can_rxmsg/7 -> CANRxField5/1  "result_volt_ch1_system_error"
  raptor_can_rxmsg/6 -> CANRxField4/1  "result_volt_ch1_mux_id"
  CANRxField/1 -> Bus Creator/2
  CANRxField1/1 -> Bus Creator/3
  CANRxField2/1 -> Bus Creator/4
  CANRxField3/1 -> Bus Creator/5
  CANRxField4/1 -> Bus Creator/6
  CANRxField5/1 -> Bus Creator/7
  CANRxField6/1 -> Bus Creator/8

== system VCMGCM1962020b_v2/Fgnd/Sensors/CAN/Other/Cooling Pump 1/MsgName ==
  DiagEnbl : Inport
  Bus Creator : BusCreator  Inputs=9
  CANRxField{,1..4} (5 alike) : Blocks_lib/CANRxField  typ='uint8'  custom=on  custom_nam=[nam '---']  custom_units='---'
  CANRxField(J1939) : Blocks_lib/CANRxField(J1939)  typ='double'  custom=on  custom_nam=[nam '---']  custom_units='---'
  CANRxField(J1939)1 : Blocks_lib/CANRxField(J1939)  typ='double'  custom=on  custom_nam=[nam '---']  custom_units='---'
  CANRxField(J1939)2 : Blocks_lib/CANRxField(J1939)  typ='double'  custom=on  custom_nam=[nam '---']  custom_units='---'
  CANRxMsgStatus : Blocks_lib/CANRxMsgStatus  samptime=samptime  custom=on  custom_nam=[nam '---']  msgnam=CoolPump1EAPMCPS
  Header : Blocks_lib/Header  width=Landscape  addtext=''
  Terminator{,1..4} (5 alike) : Terminator
  raptor_can_rxmsg : Raptor_lib/CAN/raptor_can_rxmsg  canDefinition=struct('dbcFile', 'EMPMotorController.dbc','message', 'EAPMCPS','comment', '','signals', {{'EnableStatus','ControllerStatusReason','ControllerCommand','MotorSpeed','ControlTemperature','Power','ServiceIndicator','OperatingStatus'}},'enabled', [ 1 1 1 1 1 1 1 1;],'canBus', 'bus','messageID', [ 419167744;],'idMask', [ 536870656;],'payloadMask', [],'payloadValue', [],'period', [ 0;],'mailbox', 'msgnam','queueSize', [ 1;],'label', [ 1;],'ver', [ 2;],'showID', [ 0;],'showRaw', [ 1;],'fill', [ 0;],'editID', [ 0;],'signalOrder', [ 3;],'signalAscDes', [ 1;])  canBus=bus  mailbox=msgnam  payloadMask=[]  payloadValue=[]  idMask=hex2dec('1FFFFF00')  queueSize=1  showID=0  label=1  fill=0  id=419167744  showRaw=1  showAge=1  signalOrder=3  signalInfo={{struct('Name', 'EnableStatus','Startbit', [ 0;],'SignalSize', [ 2;],'ByteOrder', 'LittleEndian','ValueType', 'UNSIGNED','Class', 'uint8','Signed', [ 0;],'Factor', [ 1;],'Offset', [ 0;],'Min', [ 0;],'Max', [ 3;],'Units', '','Comment', '','StartBit', [ 0;]),struct('Name', 'ControllerStatusReason','Startbit', [ 0;],'SignalSize', [ 4;],'ByteOrder', 'LittleEndian','ValueType', 'UNSIGNED','Class', 'uint8','Signed', [ 0;],'Factor', [ 1;],'Offset', [ 0;],'Min', [ 0;],'Max', [ 15;],'Units', '','Comment', '','StartBit', [ 2;]),struct('Name', 'ControllerCommand','Startbit', [ 0;],'SignalSize', [ 2;],'ByteOrder', 'LittleEndian','ValueType', 'UNSIGNED','Class', 'uint8','Signed', [ 0;],'Factor', [ 1;],'Offset', [ 0;],'Min', [ 0;],'Max', [ 3;],'Units', '','Comment', '','StartBit', [ 6;]),struct('Name', 'MotorSpeed','Startbit', [ 0;],'SignalSize', [ 16;],'ByteOrder', 'LittleEndian','ValueType', 'UNSIGNED','Class', 'uint16','Signed', [ 0;],'Factor', [ 0.5;],'Offset', [ 0;],'Min', [ 0;],'Max', [ 32127.5;],'Units', 'rpm','Comment', '','StartBit', [ 8;]),struct('Name', 'ControlTemperature','Startbit', [ 0;],'SignalSize', [ 16;],'ByteOrder', 'LittleEndian','ValueType', 'UNSIGNED','Class', 'uint16','Signed', [ 0;],'Factor', [ 0.03125;],'Offset', [ -237;],'Min', [ -273;],'Max', [ 1734.9688;],'Units', 'degC','Comment', '','StartBit', [ 24;]),struct('Name', 'Power','Startbit', [ 0;],'SignalSize', [ 16;],'ByteOrder', 'LittleEndian','ValueType', 'UNSIGNED','Class', 'uint16','Signed', [ 0;],'Factor', [ 0.5;],'Offset', [ 0;],'Min', [ 0;],'Max', [ 1734.9688;],'Units', 'W','Comment', '','StartBit', [ 40;]),struct('Name', 'ServiceIndicator','Startbit', [ 0;],'SignalSize', [ 2;],'ByteOrder', 'LittleEndian','ValueType', 'UNSIGNED','Class', 'uint8','Signed', [ 0;],'Factor', [ 1;],'Offset', [ 0;],'Min', [ 0;],'Max', [ 3;],'Units', '','Comment', '','StartBit', [ 56;]),struct('Name', 'OperatingStatus','Startbit', [ 0;],'SignalSize', [ 2;],'ByteOrder', 'LittleEndian','ValueType', 'UNSIGNED','Class', 'uint8','Signed', [ 0;],'Factor', [ 1;],'Offset', [ 0;],'Min', [ 0;],'Max', [ 3;],'Units', '','Comment', '','StartBit', [ 58;])}}
      settings: SourceProductName=Raptor
  Data : Outport  VectorParamsAs1DForOutWhenUnconnected=off
  wires:
  Bus Creator/1 -> Data/1  "MsgName"
  raptor_can_rxmsg/3 -> Terminator/1  "EnableStatus_raw"
  raptor_can_rxmsg/5 -> Terminator1/1  "ControllerStatusReason_raw"
  raptor_can_rxmsg/7 -> Terminator2/1  "ControllerCommand_raw"
  raptor_can_rxmsg/17 -> Terminator4/1  "OperatingStatus_raw"
  raptor_can_rxmsg/15 -> Terminator3/1  "ServiceIndicator_raw"
  raptor_can_rxmsg/1 -> CANRxMsgStatus/2  "Age"
  CANRxField(J1939)1/1 -> Bus Creator/6
  CANRxField(J1939)/1 -> Bus Creator/5
  CANRxField(J1939)2/1 -> Bus Creator/7
  CANRxField3/1 -> Bus Creator/8
  CANRxField4/1 -> Bus Creator/9
  CANRxField2/1 -> Bus Creator/4
  CANRxField1/1 -> Bus Creator/3
  CANRxMsgStatus/1 -> Bus Creator/1
  CANRxField/1 -> Bus Creator/2
  raptor_can_rxmsg/2 -> CANRxField/1  "EnableStatus"
  raptor_can_rxmsg/4 -> CANRxField1/1  "ControllerStatusReason"
  raptor_can_rxmsg/6 -> CANRxField2/1  "ControllerCommand"
  raptor_can_rxmsg/14 -> CANRxField3/1  "ServiceIndicator"
  raptor_can_rxmsg/16 -> CANRxField4/1  "OperatingStatus"
  raptor_can_rxmsg/9 -> CANRxField(J1939)/2  "MotorSpeed_raw"
  raptor_can_rxmsg/11 -> CANRxField(J1939)1/2  "ControlTemperature_raw"
  raptor_can_rxmsg/13 -> CANRxField(J1939)2/2  "Power_raw"
  raptor_can_rxmsg/8 -> CANRxField(J1939)/1  "MotorSpeed"
  raptor_can_rxmsg/10 -> CANRxField(J1939)1/1  "ControlTemperature"
  raptor_can_rxmsg/12 -> CANRxField(J1939)2/1  "Power"
  DiagEnbl/1 -> CANRxMsgStatus/1

== system VCMGCM1962020b_v2/Fgnd/Sensors/CAN/Other/Cooling Pump 1/Set Rx IDs ==
  f : TriggerPort  TriggerType=function-call  VariantControl=(inherit)  PortDimensions=1
  Constant : Constant  Value=hex2dec('FF')  OutDataTypeStr=Inherit: Inherit via back propagation
  Data Type Conversion : DataTypeConversion  OutDataTypeStr=uint32
  Header : Blocks_lib/Header  width=Portrait  addtext=''
  raptor_adjustment : Raptor_lib/Data Storage/raptor_adjustment  paramName=[nam 'J1939SA']  nameSource=Parameter  initValue=0  dataType=uint8  storage=Calibration  calDispType=Number  calEnum={'False', 'True'}  calGain=1.0  calOffset=0.0  calMax=inf  calMin=-inf  calFormat=''  calUnit=''  calHelp='J1939 source address'  calAccess=1  calFunction='Sensors | CAN'  calDispHeaders=off  calColHeaders={'Col1' 'Col2' 'Col3'}  calRowHeaders={'Row1' 'Row2' 'Row3'}
      settings: SourceProductName=Raptor
  raptor_can_mailbox_properties : Raptor_lib/CAN/raptor_can_mailbox_properties  mailbox=[nam 'EAPMCPS']
      settings: SourceProductName=Raptor
  wires:
  raptor_adjustment/1 -> Data Type Conversion/1
  Constant/1 -> raptor_can_mailbox_properties/2
  Data Type Conversion/1 -> raptor_can_mailbox_properties/1

== system VCMGCM1962020b_v2/Fgnd/Sensors/CAN/Other/Cooling Pump 2/MsgName ==
  DiagEnbl : Inport
  Bus Creator : BusCreator  Inputs=9
  CANRxField{,1..4} (5 alike) : Blocks_lib/CANRxField  typ='uint8'  custom=on  custom_nam=[nam '---']  custom_units='---'
  CANRxField(J1939) : Blocks_lib/CANRxField(J1939)  typ='double'  custom=on  custom_nam=[nam '---']  custom_units='---'
  CANRxField(J1939)1 : Blocks_lib/CANRxField(J1939)  typ='double'  custom=on  custom_nam=[nam '---']  custom_units='---'
  CANRxField(J1939)2 : Blocks_lib/CANRxField(J1939)  typ='double'  custom=on  custom_nam=[nam '---']  custom_units='---'
  CANRxMsgStatus : Blocks_lib/CANRxMsgStatus  samptime=samptime  custom=on  custom_nam=[nam '---']  msgnam=CoolPump2EAPMCPS
  Header : Blocks_lib/Header  width=Landscape  addtext=''
  Terminator{,1..4} (5 alike) : Terminator
  raptor_can_rxmsg : Raptor_lib/CAN/raptor_can_rxmsg  canDefinition=struct('dbcFile', 'EMPMotorController.dbc','message', 'EAPMCPS','comment', '','signals', {{'EnableStatus','ControllerStatusReason','ControllerCommand','MotorSpeed','ControlTemperature','Power','ServiceIndicator','OperatingStatus'}},'enabled', [ 1 1 1 1 1 1 1 1;],'canBus', 'bus','messageID', [ 419167744;],'idMask', [ 536870656;],'payloadMask', [],'payloadValue', [],'period', [ 0;],'mailbox', 'msgnam','queueSize', [ 1;],'label', [ 1;],'ver', [ 2;],'showID', [ 0;],'showRaw', [ 1;],'fill', [ 0;],'editID', [ 0;],'signalOrder', [ 3;],'signalAscDes', [ 1;])  canBus=bus  mailbox=msgnam  payloadMask=[]  payloadValue=[]  idMask=hex2dec('1FFFFF00')  queueSize=1  showID=0  label=1  fill=0  id=419167744  showRaw=1  showAge=1  signalOrder=3  signalInfo={{struct('Name', 'EnableStatus','Startbit', [ 0;],'SignalSize', [ 2;],'ByteOrder', 'LittleEndian','ValueType', 'UNSIGNED','Class', 'uint8','Signed', [ 0;],'Factor', [ 1;],'Offset', [ 0;],'Min', [ 0;],'Max', [ 3;],'Units', '','Comment', '','StartBit', [ 0;]),struct('Name', 'ControllerStatusReason','Startbit', [ 0;],'SignalSize', [ 4;],'ByteOrder', 'LittleEndian','ValueType', 'UNSIGNED','Class', 'uint8','Signed', [ 0;],'Factor', [ 1;],'Offset', [ 0;],'Min', [ 0;],'Max', [ 15;],'Units', '','Comment', '','StartBit', [ 2;]),struct('Name', 'ControllerCommand','Startbit', [ 0;],'SignalSize', [ 2;],'ByteOrder', 'LittleEndian','ValueType', 'UNSIGNED','Class', 'uint8','Signed', [ 0;],'Factor', [ 1;],'Offset', [ 0;],'Min', [ 0;],'Max', [ 3;],'Units', '','Comment', '','StartBit', [ 6;]),struct('Name', 'MotorSpeed','Startbit', [ 0;],'SignalSize', [ 16;],'ByteOrder', 'LittleEndian','ValueType', 'UNSIGNED','Class', 'uint16','Signed', [ 0;],'Factor', [ 0.5;],'Offset', [ 0;],'Min', [ 0;],'Max', [ 32127.5;],'Units', 'rpm','Comment', '','StartBit', [ 8;]),struct('Name', 'ControlTemperature','Startbit', [ 0;],'SignalSize', [ 16;],'ByteOrder', 'LittleEndian','ValueType', 'UNSIGNED','Class', 'uint16','Signed', [ 0;],'Factor', [ 0.03125;],'Offset', [ -237;],'Min', [ -273;],'Max', [ 1734.9688;],'Units', 'degC','Comment', '','StartBit', [ 24;]),struct('Name', 'Power','Startbit', [ 0;],'SignalSize', [ 16;],'ByteOrder', 'LittleEndian','ValueType', 'UNSIGNED','Class', 'uint16','Signed', [ 0;],'Factor', [ 0.5;],'Offset', [ 0;],'Min', [ 0;],'Max', [ 1734.9688;],'Units', 'W','Comment', '','StartBit', [ 40;]),struct('Name', 'ServiceIndicator','Startbit', [ 0;],'SignalSize', [ 2;],'ByteOrder', 'LittleEndian','ValueType', 'UNSIGNED','Class', 'uint8','Signed', [ 0;],'Factor', [ 1;],'Offset', [ 0;],'Min', [ 0;],'Max', [ 3;],'Units', '','Comment', '','StartBit', [ 56;]),struct('Name', 'OperatingStatus','Startbit', [ 0;],'SignalSize', [ 2;],'ByteOrder', 'LittleEndian','ValueType', 'UNSIGNED','Class', 'uint8','Signed', [ 0;],'Factor', [ 1;],'Offset', [ 0;],'Min', [ 0;],'Max', [ 3;],'Units', '','Comment', '','StartBit', [ 58;])}}
      settings: SourceProductName=Raptor
  Data : Outport  VectorParamsAs1DForOutWhenUnconnected=off
  wires:
  DiagEnbl/1 -> CANRxMsgStatus/1
  raptor_can_rxmsg/12 -> CANRxField(J1939)2/1  "Power"
  raptor_can_rxmsg/10 -> CANRxField(J1939)1/1  "ControlTemperature"
  raptor_can_rxmsg/8 -> CANRxField(J1939)/1  "MotorSpeed"
  raptor_can_rxmsg/13 -> CANRxField(J1939)2/2  "Power_raw"
  raptor_can_rxmsg/11 -> CANRxField(J1939)1/2  "ControlTemperature_raw"
  raptor_can_rxmsg/9 -> CANRxField(J1939)/2  "MotorSpeed_raw"
  raptor_can_rxmsg/16 -> CANRxField4/1  "OperatingStatus"
  raptor_can_rxmsg/14 -> CANRxField3/1  "ServiceIndicator"
  raptor_can_rxmsg/6 -> CANRxField2/1  "ControllerCommand"
  raptor_can_rxmsg/4 -> CANRxField1/1  "ControllerStatusReason"
  raptor_can_rxmsg/2 -> CANRxField/1  "EnableStatus"
  CANRxField/1 -> Bus Creator/2
  CANRxMsgStatus/1 -> Bus Creator/1
  CANRxField1/1 -> Bus Creator/3
  CANRxField2/1 -> Bus Creator/4
  CANRxField4/1 -> Bus Creator/9
  CANRxField3/1 -> Bus Creator/8
  CANRxField(J1939)2/1 -> Bus Creator/7
  CANRxField(J1939)/1 -> Bus Creator/5
  CANRxField(J1939)1/1 -> Bus Creator/6
  raptor_can_rxmsg/1 -> CANRxMsgStatus/2  "Age"
  raptor_can_rxmsg/15 -> Terminator3/1  "ServiceIndicator_raw"
  raptor_can_rxmsg/17 -> Terminator4/1  "OperatingStatus_raw"
  raptor_can_rxmsg/7 -> Terminator2/1  "ControllerCommand_raw"
  raptor_can_rxmsg/5 -> Terminator1/1  "ControllerStatusReason_raw"
  raptor_can_rxmsg/3 -> Terminator/1  "EnableStatus_raw"
  Bus Creator/1 -> Data/1  "MsgName"

== system VCMGCM1962020b_v2/Fgnd/Sensors/CAN/Other/Cooling Pump 2/Set Rx IDs ==
  f : TriggerPort  TriggerType=function-call  VariantControl=(inherit)  PortDimensions=1
  Constant : Constant  Value=hex2dec('FF')  OutDataTypeStr=Inherit: Inherit via back propagation
  Data Type Conversion : DataTypeConversion  OutDataTypeStr=uint32
  Header : Blocks_lib/Header  width=Portrait  addtext=''
  raptor_adjustment : Raptor_lib/Data Storage/raptor_adjustment  paramName=[nam 'J1939SA']  nameSource=Parameter  initValue=0  dataType=uint8  storage=Calibration  calDispType=Number  calEnum={'False', 'True'}  calGain=1.0  calOffset=0.0  calMax=inf  calMin=-inf  calFormat=''  calUnit=''  calHelp='J1939 source address'  calAccess=1  calFunction='Sensors | CAN'  calDispHeaders=off  calColHeaders={'Col1' 'Col2' 'Col3'}  calRowHeaders={'Row1' 'Row2' 'Row3'}
      settings: SourceProductName=Raptor
  raptor_can_mailbox_properties : Raptor_lib/CAN/raptor_can_mailbox_properties  mailbox=[nam 'EAPMCPS']
      settings: SourceProductName=Raptor
  wires:
  Data Type Conversion/1 -> raptor_can_mailbox_properties/1
  Constant/1 -> raptor_can_mailbox_properties/2
  raptor_adjustment/1 -> Data Type Conversion/1

== system VCMGCM1962020b_v2/Fgnd/Sensors/CAN/Other/EPAS/EPASG7GenericFdbk0 ==
  DiagEnbl : Inport
  Bus Creator : BusCreator  Inputs=5
  CANRxField{,1..3} (4 alike) : Blocks_lib/CANRxField  typ='double'  custom=off  custom_nam=[nam '---']  custom_units='---'
  CANRxMsgStatus : Blocks_lib/CANRxMsgStatus  samptime=samptime  custom=on  custom_nam=[nam '---']  msgnam=EPASG7GenericFdbk0
  Header : Blocks_lib/Header  width=Landscape  addtext=''
  raptor_can_rxmsg : Raptor_lib/CAN/raptor_can_rxmsg  canDefinition=struct('dbcFile', 'EPAS_G7GenericExternal.dbc','message', 'G7GenericFdbk0','comment', '','signals', {{'FDBK0_TorqueIn','FDBK0_AssistCommand','FDBK0_Temperature','FDBK0_QAxisCurrent'}},'enabled', [ 1 1 1 1;],'scaled', [ 1 1 1 1;],'canBus', 'bus','messageID', [ 419365139;],'idMask', [ 536870911;],'payloadMask', [],'payloadValue', [],'period', [ 0;],'mailbox', '[]','queueSize', [ 1;],'label', [ 1;],'ver', [ 2;],'showID', [ 0;],'showRaw', [ 0;],'fill', [ 0;],'editID', [ 0;],'signalOrder', [ 3;],'signalAscDes', [ 1;])  canBus=bus  mailbox=[]  payloadMask=[]  payloadValue=[]  idMask=hex2dec('1FFFFFFF')  queueSize=1  showID=0  label=1  fill=0  id=419365139  showRaw=0  showAge=1  signalOrder=3  signalInfo={{struct('Name', 'FDBK0_TorqueIn','Startbit', [ 0;],'SignalSize', [ 16;],'ByteOrder', 'LittleEndian','ValueType', 'UNSIGNED','Class', 'uint16','Signed', [ 0;],'Factor', [ 0.1;],'Offset', [ -3200;],'Min', [ -3200;],'Max', [ 3200;],'Units', 'Nm','Comment', '','StartBit', [ 0;]),struct('Name', 'FDBK0_AssistCommand','Startbit', [ 0;],'SignalSize', [ 16;],'ByteOrder', 'LittleEndian','ValueType', 'UNSIGNED','Class', 'uint16','Signed', [ 0;],'Factor', [ 0.1;],'Offset', [ -3200;],'Min', [ -3200;],'Max', [ 3200;],'Units', '%','Comment', '','StartBit', [ 16;]),struct('Name', 'FDBK0_Temperature','Startbit', [ 0;],'SignalSize', [ 8;],'ByteOrder', 'LittleEndian','ValueType', 'UNSIGNED','Class', 'uint8','Signed', [ 0;],'Factor', [ 1;],'Offset', [ -40;],'Min', [ -40;],'Max', [ 215;],'Units', 'C','Comment', '','StartBit', [ 56;]),struct('Name', 'FDBK0_QAxisCurrent','Startbit', [ 0;],'SignalSize', [ 16;],'ByteOrder', 'LittleEndian','ValueType', 'UNSIGNED','Class', 'uint16','Signed', [ 0;],'Factor', [ 0.0038147;],'Offset', [ -125;],'Min', [ -125;],'Max', [ 124.9962;],'Units', 'Amps','Comment', '','StartBit', [ 32;])}}
      settings: SourceProductName=Raptor
  Data : Outport  VectorParamsAs1DForOutWhenUnconnected=off
  wires:
  Bus Creator/1 -> Data/1  "EPASG7GenericFdbk0"
  raptor_can_rxmsg/2 -> CANRxField/1  "FDBK0_TorqueIn"
  CANRxMsgStatus/1 -> Bus Creator/1
  CANRxField/1 -> Bus Creator/2
  DiagEnbl/1 -> CANRxMsgStatus/1
  raptor_can_rxmsg/1 -> CANRxMsgStatus/2  "Age"
  raptor_can_rxmsg/3 -> CANRxField1/1  "FDBK0_AssistCommand"
  raptor_can_rxmsg/4 -> CANRxField2/1  "FDBK0_Temperature"
  raptor_can_rxmsg/5 -> CANRxField3/1  "FDBK0_QAxisCurrent"
  CANRxField1/1 -> Bus Creator/3
  CANRxField2/1 -> Bus Creator/4
  CANRxField3/1 -> Bus Creator/5

== system VCMGCM1962020b_v2/Fgnd/Sensors/CAN/Other/EPAS/EPASG7GenericFdbk1 ==
  DiagEnbl : Inport
  Bus Creator : BusCreator  Inputs=3
  CANRxField : Blocks_lib/CANRxField  typ='double'  custom=off  custom_nam=[nam '---']  custom_units='---'
  CANRxField1 : Blocks_lib/CANRxField  typ='double'  custom=off  custom_nam=[nam '---']  custom_units='---'
  CANRxMsgStatus : Blocks_lib/CANRxMsgStatus  samptime=samptime  custom=on  custom_nam=[nam '---']  msgnam=EPASG7GenericFdbk1
  Header : Blocks_lib/Header  width=Landscape  addtext=''
  raptor_can_rxmsg : Raptor_lib/CAN/raptor_can_rxmsg  canDefinition=struct('dbcFile', 'EPAS_G7GenericExternal.dbc','message', 'G7GenericFdbk1','comment', '','signals', {{'FDBK1_QAxisCurrent','FDBK1_Position'}},'enabled', [ 1 1;],'scaled', [ 1 1;],'canBus', 'bus','messageID', [ 419365395;],'idMask', [ 536870911;],'payloadMask', [],'payloadValue', [],'period', [ 0;],'mailbox', '[]','queueSize', [ 1;],'label', [ 1;],'ver', [ 2;],'showID', [ 0;],'showRaw', [ 0;],'fill', [ 0;],'editID', [ 0;],'signalOrder', [ 3;],'signalAscDes', [ 1;])  canBus=bus  mailbox=[]  payloadMask=[]  payloadValue=[]  idMask=hex2dec('1FFFFFFF')  queueSize=1  showID=0  label=1  fill=0  id=419365395  showRaw=0  showAge=1  signalOrder=3  signalInfo={{struct('Name', 'FDBK1_QAxisCurrent','Startbit', [ 0;],'SignalSize', [ 32;],'ByteOrder', 'LittleEndian','ValueType', 'SIGNED','Class', 'int32','Signed', [ 1;],'Factor', [ 9.5367e-07;],'Offset', [ 0;],'Min', [ -2048;],'Max', [ 2048;],'Units', 'Amps','Comment', '','StartBit', [ 32;]),struct('Name', 'FDBK1_Position','Startbit', [ 0;],'SignalSize', [ 32;],'ByteOrder', 'LittleEndian','ValueType', 'SIGNED','Class', 'int32','Signed', [ 1;],'Factor', [ 9.5367e-07;],'Offset', [ 0;],'Min', [ -2048;],'Max', [ 2048;],'Units', 'Revs','Comment', '','StartBit', [ 0;])}}
      settings: SourceProductName=Raptor
  Data : Outport  VectorParamsAs1DForOutWhenUnconnected=off
  wires:
  CANRxField1/1 -> Bus Creator/3
  raptor_can_rxmsg/3 -> CANRxField1/1  "FDBK1_Position"
  raptor_can_rxmsg/1 -> CANRxMsgStatus/2  "Age"
  DiagEnbl/1 -> CANRxMsgStatus/1
  CANRxField/1 -> Bus Creator/2
  CANRxMsgStatus/1 -> Bus Creator/1
  raptor_can_rxmsg/2 -> CANRxField/1  "FDBK1_QAxisCurrent"
  Bus Creator/1 -> Data/1  "EPASG7GenericFdbk1"
